simulink model "Mdl_Sample"  (R2020b)
settings: Solver=FixedStepAuto  StartTime=0.0  StopTime=1.23  FixedStep=0.01  RelTol=1e-3
undefined symbols (not defined in the file or in its folder): sigbuilder_block
settings Model: Creator=amimoto  LastModifiedBy=amimoto

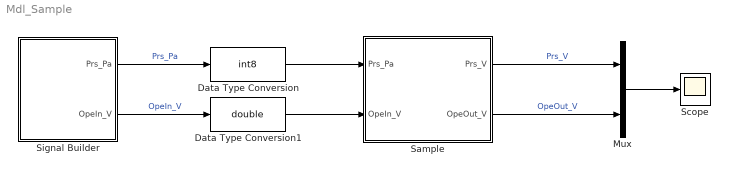
== system Mdl_Sample ==
  Data Type Conversion : DataTypeConversion  OutDataTypeStr=int8
  Data Type Conversion1 : DataTypeConversion  OutDataTypeStr=double
  Mux : Mux  Inputs=2
  Sample : Subsystem
  Scope : Scope
  Signal Builder : Subsystem  Tag=STV Subsys  LoadFcn=sigbuilder_block('load');  StartFcn=sigbuilder_block('start');  StopFcn=sigbuilder_block('stop');  ClipboardFcn=sigbuilder_block('clipboard');  mask(Sigbuilder block){tuvar=[0:10]}
      mask help: Simulink:masks:SigbuilderBlock_MD
      mask init:
      | if ~strcmp(get_param(bdroot(gcbh),'SimulationStatus'),'stopped') tuvar = sigbuilder_block('maskInit'); end
      settings: CopyFcn=sigbuilder_block('copy');  DeleteFcn=sigbuilder_block('delete');  ModelCloseFcn=sigbuilder_block('modelClose');  PreSaveFcn=sigbuilder_block('preSave');  PauseFcn=sigbuilder_block('pause');  ContinueFcn=sigbuilder_block('continue');  NameChangeFcn=sigbuilder_block('namechange');  OpenFcn=sigbuilder_block('open',[437.6 199.2 550.4 400 ]);  CloseFcn=sigbuilder_block('close');
      mask Display: plot(0, 0, 100, 100,[2, 2, 32, 32, 2], [68, 8, 8, 68, 68],[32, 2], [38, 38], [32, 19, 2],[53, 60, 44], [32, 17, 17, 2],[16, 16, 31, 31]);txt = getActiveGroup(gcbh);text(2, 100, txt,'verticalAlignment', 'top');
  wires:
  Signal Builder/1(Prs_Pa) -> Data Type Conversion/1  "Prs_Pa"
  Signal Builder/2(OpeIn_V) -> Data Type Conversion1/1  "OpeIn_V"
  Sample/1(Prs_V) -> Mux/1  "Prs_V"
  Sample/2(OpeOut_V) -> Mux/2  "OpeOut_V"
  Data Type Conversion/1 -> Sample/1(Prs_Pa)
  Data Type Conversion1/1 -> Sample/2(OpeIn_V)
  Mux/1 -> Scope/1

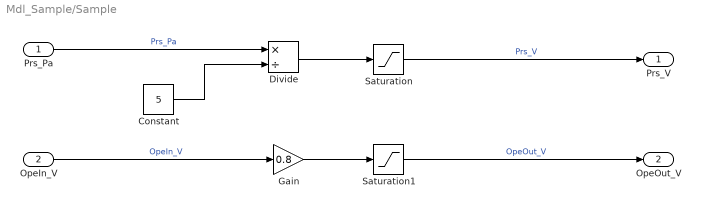
== system Mdl_Sample/Sample ==
  Prs_Pa : Inport
  OpeIn_V : Inport  Port=2
  Constant : Constant  Value=5
  Divide : Product  Inputs=*/
  Gain : Gain  Gain=0.8
  Saturation : Saturate  UpperLimit=5  LowerLimit=1
  Saturation1 : Saturate  UpperLimit=4  LowerLimit=1
  Prs_V : Outport
  OpeOut_V : Outport  Port=2
  wires:
  Saturation1/1 -> OpeOut_V/1  "OpeOut_V"
  Gain/1 -> Saturation1/1
  Divide/1 -> Saturation/1
  Prs_Pa/1 -> Divide/1  "Prs_Pa"
  OpeIn_V/1 -> Gain/1  "OpeIn_V"
  Constant/1 -> Divide/2
  Saturation/1 -> Prs_V/1  "Prs_V"

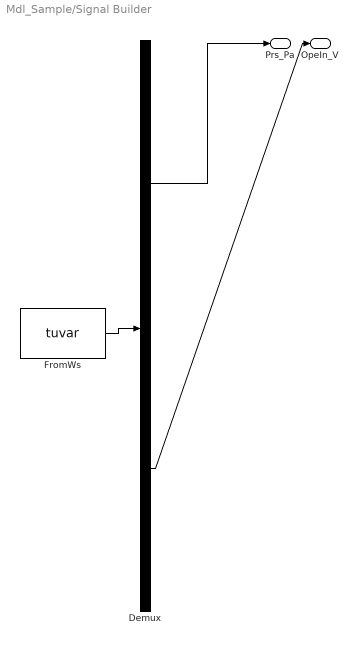
== system Mdl_Sample/Signal Builder ==
  Demux : Demux  Tag=STV Demux  Outputs=2
      settings: DisplayOption=none
  FromWs : FromWorkspace  Tag=STV FromWs  VariableName=tuvar
      SigBuilderData=|
      | common.afterFinalStr = 'Extrapolate'
      | common.sampleTime = 0
      | dataSet.timeRange = [0 1.23]
      | dataSet.name = 'Sheet1'
      | sbobj.Name = 'Signal Builder'
      | sbobj.Groups.Name = 'Sheet1'
      | sbobj.Groups.Signals(1).Name = 'Prs_Pa'
      | sbobj.Groups.Signals(1).XData = [0 0.01 0.02 0.03 0.04 0.05 0.06 0.07 0.08 0.09 0.1 0.11 0.12 0.13 0.14 0.15 0.16 0.17 0.18 0.19 0.2 0.21 0.22 0.23 0.24 0.25 0.26 0.27 0.28 0.29 0.3 0.31 0.32 0.33 0.34 0.35 0.36 0.37 0.38 0.39 0.4 0.41 0.42 0.43 0.44 0.45 0.46 0.47 0.48 0.49 0.5 0.51 0.52 0.53 0.54 0.55 0.56 0.57 0.58 0.59 0.6 0.61 0.62 0.63 0.64 0.65 0.66 0.67 0.68 0.69 0.7 0.71 0.72 0.73 0.74 0.75 0.76 0.77 0.78 0.79 0.8 0.81 0.82 0.83 0.84 0.85 0.86 0.87 0.88 0.89 0.9 0.91 0.92 0.93 0.94 0.95 0.96 0.97 0.98 0.99 1 1.01 1.02 1.03 1.04 1.05 1.06 1.07 1.08 1.09 1.1 1.11 1.12 1.13 1.14 1.15 1.16 1.17 1.18 1.19 1.2 1.21 1.22 1.23]
      | sbobj.Groups.Signals(1).YData = [0 0 0 0 1 1 1 1 2 2 2 2 3 3 3 3 4 4 4 4 5 5 5 5 6 6 6 6 7 7 7 7 8 8 8 8 9 9 9 9 10 10 10 10 11 11 11 11 12 12 12 12 13 13 13 13 14 14 14 14 15 15 15 15 16 16 16 16 17 17 17 17 18 18 18 18 19 19 19 19 20 20 20 20 21 21 21 21 22 22 22 22 23 23 23 23 24 24 24 24 25 25 25 25 26 26 26 26 27 27 27 27 28 28 28 28 29 29 29 29 30 30 30 30]
      | sbobj.Groups.Signals(2).Name = 'OpeIn_V'
      | sbobj.Groups.Signals(2).XData = [0 0.01 0.02 0.03 0.04 0.05 0.06 0.07 0.08 0.09 0.1 0.11 0.12 0.13 0.14 0.15 0.16 0.17 0.18 0.19 0.2 0.21 0.22 0.23 0.24 0.25 0.26 0.27 0.28 0.29 0.3 0.31 0.32 0.33 0.34 0.35 0.36 0.37 0.38 0.39 0.4 0.41 0.42 0.43 0.44 0.45 0.46 0.47 0.48 0.49 0.5 0.51 0.52 0.53 0.54 0.55 0.56 0.57 0.58 0.59 0.6 0.61 0.62 0.63 0.64 0.65 0.66 0.67 0.68 0.69 0.7 0.71 0.72 0.73 0.74 0.75 0.76 0.77 0.78 0.79 0.8 0.81 0.82 0.83 0.84 0.85 0.86 0.87 0.88 0.89 0.9 0.91 0.92 0.93 0.94 0.95 0.96 0.97 0.98 0.99 1 1.01 1.02 1.03 1.04 1.05 1.06 1.07 1.08 1.09 1.1 1.11 1.12 1.13 1.14 1.15 1.16 1.17 1.18 1.19 1.2 1.21 1.22 1.23]
      | sbobj.Groups.Signals(2).YData = [0 0 0 0 0.2 0.2 0.2 0.2 0.4 0.4 0.4 0.4 0.6 0.6 0.6 0.6 0.8 0.8 0.8 0.8 1 1 1 1 1.2 1.2 1.2 1.2 1.4 1.4 1.4 1.4 1.6 1.6 1.6 1.6 1.8 1.8 1.8 1.8 2 2 2 2 2.2 2.2 2.2 2.2 2.4 2.4 2.4 2.4 2.6 2.6 2.6 2.6 2.8 2.8 2.8 2.8 3 3 3 3 3.2 3.2 3.2 3.2 3.4 3.4 3.4 3.4 3.6 3.6 3.6 3.6 3.8 3.8 3.8 3.8 4 4 4 4 4.2 4.2 4.2 4.2 4.4 4.4 4.4 4.4 4.6 4.6 4.6 4.6 4.8 4.8 4.8 4.8 5 5 5 5 5.2 5.2 5.2 5.2 5.4 5.4 5.4 5.4 5.6 5.6 5.6 5.6 5.8 5.8 5.8 5.8 6 6 6 6]
      | sbobj.Groups.TimeRange = [0 1.23]
  Prs_Pa : Outport  Tag=STV Outport
  OpeIn_V : Outport  Tag=STV Outport  Port=2
  wires:
  Demux/1 -> Prs_Pa/1
  FromWs/1 -> Demux/1
  Demux/2 -> OpeIn_V/1
